simulink model "Mdl_Speed"  (R2024b)
settings: Solver=FixedStepDiscrete  StartTime=0.0  StopTime=10.0  FixedStep=0.1  RelTol=1e-3  EnableMultiTasking=on
values from neighbouring files (symbols this model uses):
  AI_TEMP_ADC_COUNT_1586 = mpt.Parameter    [Mdl_Speed_lookup.m]
  AI_TEMP_ADC_COUNT_1727 = mpt.Parameter    [Mdl_Speed_lookup.m]
  AI_TEMP_ADC_COUNT_1792 = mpt.Parameter    [Mdl_Speed_lookup.m]
  AI_TEMP_ADC_COUNT_1891 = mpt.Parameter    [Mdl_Speed_lookup.m]
  C_ADR = mpt.Parameter    [Mdl_Speed_lookup.m]
  C_CANADA = mpt.Parameter    [Mdl_Speed_lookup.m]
  C_EUROPE = mpt.Parameter    [Mdl_Speed_lookup.m]
  C_KOREA = mpt.Parameter    [Mdl_Speed_lookup.m]
  C_MEXICO = mpt.Parameter    [Mdl_Speed_lookup.m]
  C_UK = mpt.Parameter    [Mdl_Speed_lookup.m]
  C_USA = mpt.Parameter    [Mdl_Speed_lookup.m]
  eSP_ADR = mpt.Parameter    [Speed_Table_Type_param.m]
  eSP_CANADA = mpt.Parameter    [Speed_Table_Type_param.m]
  eSP_ECE = mpt.Parameter    [Speed_Table_Type_param.m]
  eSP_EUROPE = mpt.Parameter    [Speed_Table_Type_param.m]
  eSP_KOREA_FMVSS = mpt.Parameter    [Speed_Table_Type_param.m]
  eSP_KOREA_UN_R = mpt.Parameter    [Speed_Table_Type_param.m]
  eSP_MEXICO_FMVSS = mpt.Parameter    [Speed_Table_Type_param.m]
  eSP_MEXICO_UN_R = mpt.Parameter    [Speed_Table_Type_param.m]
  eSP_UK = mpt.Parameter    [Speed_Table_Type_param.m]
  eSP_USA = mpt.Parameter    [Speed_Table_Type_param.m]
  INDEX_MCUID0262 = mpt.Parameter    [Mdl_Speed_lookup.m]
  INDEX_MCUID0263 = mpt.Parameter    [Mdl_Speed_lookup.m]
  Initial_data = mpt.Parameter    [Mdl_Speed_lookup.m]
  MCUID0809 = mpt.Parameter    [Mdl_Speed_DD.m]
  MCUID0810 = mpt.Parameter    [Mdl_Speed_DD.m]
  MCUID_MAX_VAL = mpt.Parameter    [Mdl_Speed_lookup.m]
  MIN_SPEED_VALUE = mpt.Parameter    [Mdl_Speed_lookup.m]
  RESOLUTION_VAL_100 = mpt.Parameter    [Mdl_Speed_lookup.m]
  RESOLUTION_VAL_103 = mpt.Parameter    [Mdl_Speed_lookup.m]
  RESOLUTION_VAL_50 = mpt.Parameter    [Mdl_Speed_lookup.m]
  RESOLUTION_VAL_64 = mpt.Parameter    [Mdl_Speed_lookup.m]
  RESOLUTION_VAL_MINUS_100 = mpt.Parameter    [Mdl_Speed_lookup.m]
  SPEED_AVG_REF = mpt.Parameter    [Mdl_Speed_lookup.m]
  SPEED_CHECK_VALUE_ONE = mpt.Parameter    [Mdl_Speed_lookup.m]
  SPEED_UPDATE_0_28S = mpt.Parameter    [Mdl_Speed_lookup.m]
  SPEED_UPDATE_0_5S = mpt.Parameter    [Mdl_Speed_lookup.m]
  SPEED_UPDATE_1_5S = mpt.Parameter    [Mdl_Speed_lookup.m]
  SPEED_UPDATE_1S = mpt.Parameter    [Mdl_Speed_lookup.m]
  SPEED_ZERO = mpt.Parameter    [Mdl_Speed_lookup.m]
  VAL_ONE = mpt.Parameter    [Mdl_Speed_lookup.m]
  VAL_ZERO = mpt.Parameter    [Mdl_Speed_lookup.m]
undefined symbols (not defined in the file or in its folder): Arr_u8_100_type_instance, Arr_u8_1024_type_instance, Arr_u8_10_type_instance, Arr_u8_128_type_instance, Arr_u8_16_type_instance, Arr_u8_17_type_instance, Arr_u8_2048_type_instance, Arr_u8_256_type_instance, Arr_u8_32_type_instance, Arr_u8_3_type_instance, Arr_u8_46_type_instance, Arr_u8_48_type_instance, Arr_u8_61_type_instance, Arr_u8_64_type_instance, Arr_u8_8_type_instance, Arr_u8_9_type_instance, CLUSTER_ACTIVE, eIO_ADC_AI_TEMP_RTC, eSIGNAL_MISSING, eSIGNAL_NEVER_RECEIVED, eVehicleSpeedABSIn, IgnOff, IgnOn, IoHwAb_AdcSignalIdType_type_instance, IoHwAb_ErrorType_type_instance, pJustRcvdStatus, RxCan_SignalClearJustRcvdStatus, RxCan_SignalGetJustRcvdStatus, RxCan_SignalInvalidProcessingControl, RxCan_SignalMissingProcessingControl, RxCan_SignalNRProcessingControl, SignalId, SPEED_MAX_RESOLUTION, Status, tRxSignalId_type_instance, tRxSignalJustRcvdStatus_type_instance, tRxSignalStatus_type_instance
libraries: simulink x9
(part 2 of 3)

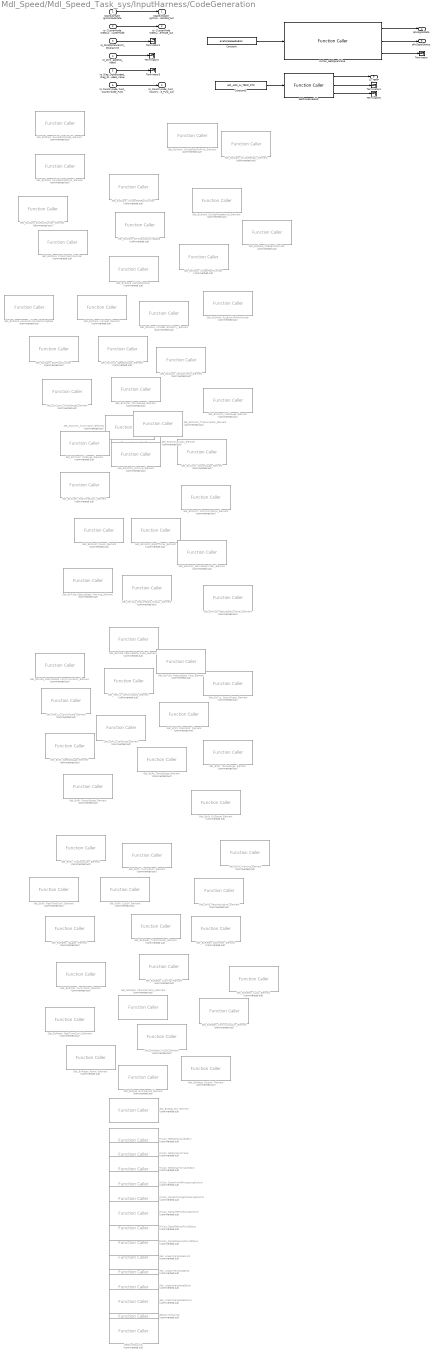
== system Mdl_Speed/Mdl_Speed_Task_sys/InputHarness/CodeGeneration ==
  rpIgnSubstate_IgnitionSubstate : Inport  OutDataTypeStr=IgntionSubstateType  PortDimensions=1
  rp_ClusterMode_WSSCurrentClusterMode : Inport  Port=2  OutDataTypeStr=ClusterModes  PortDimensions=1
  rp_DispDistanceUnit_DisplayUnit : Inport  Port=3  OutDataTypeStr=uint8  PortDimensions=1
  rp_Dcm_appStop_AppId : Inport  Port=4  OutDataTypeStr=IOCtrl_Type  PortDimensions=1
  rp_Diag_Digitalspeed_Diag_Digital_Speed_Value : Inport  Port=5  OutDataTypeStr=uint16  PortDimensions=1
  rp_Countrycode_Func_CountryCode_Func : Inport  Port=6  OutDataTypeStr=CountryCode_FuncType  PortDimensions=1
  Constant : Constant  Value=eVehicleSpeedABSIn
  Constant5 : Constant  Value=eIO_ADC_AI_TEMP_RTC  OutDataTypeStr=uint8
  GetAsyncRawAdc : FunctionCaller  Commented=on  FunctionPrototype=[AsyncRawAdc,ErrorStatus,error_status] = GetAsyncRawAdc(AdcId)  InputArgumentSpecifications=IoHwAb_AdcSignalIdType_type_instance(1)  OutputArgumentSpecifications=uint16(1) ,IoHwAb_ErrorType_type_instance(1) ,uint8(1)
  GetProcessedAdc : FunctionCaller  FunctionPrototype=[ProcessedAdc,ErrorStatus,error_status] = GetProcessedAdc(AdcId)  InputArgumentSpecifications=IoHwAb_AdcSignalIdType_type_instance(1)  OutputArgumentSpecifications=int32(1) ,IoHwAb_ErrorType_type_instance(1) ,uint8(1)
  GetSyncRawAdc : FunctionCaller  Commented=on  FunctionPrototype=[SyncRawAdc,ErrorStatus,error_status] = GetSyncRawAdc(AdcId)  InputArgumentSpecifications=IoHwAb_AdcSignalIdType_type_instance(1)  OutputArgumentSpecifications=uint16(1) ,IoHwAb_ErrorType_type_instance(1) ,uint8(1)
  Get_BsConst_Audio_Element : FunctionCaller  Commented=on  FunctionPrototype=[Ptr,error_status] = Get_BsConst_Audio_Element()  InputArgumentSpecifications=<Enter example>  OutputArgumentSpecifications=Arr_u8_128_type_instance(1) ,uint8(1)
  Get_BsConst_Communication_Element : FunctionCaller  Commented=on  FunctionPrototype=[Ptr,error_status] = Get_BsConst_Communication_Element()  InputArgumentSpecifications=<Enter example>  OutputArgumentSpecifications=Arr_u8_64_type_instance(1) ,uint8(1)
  Get_BsConst_EngOffTimer_Element : FunctionCaller  Commented=on  FunctionPrototype=[Ptr,error_status] = Get_BsConst_EngOffTimer_Element()  InputArgumentSpecifications=<Enter example>  OutputArgumentSpecifications=Arr_u8_32_type_instance(1) ,uint8(1)
  Get_BsConst_FuelGauge_Element : FunctionCaller  Commented=on  FunctionPrototype=[Ptr,error_status] = Get_BsConst_FuelGauge_Element()  InputArgumentSpecifications=<Enter example>  OutputArgumentSpecifications=Arr_u8_128_type_instance(1) ,uint8(1)
  Get_BsConst_Illumination_Element : FunctionCaller  Commented=on  FunctionPrototype=[Ptr,error_status] = Get_BsConst_Illumination_Element()  InputArgumentSpecifications=<Enter example>  OutputArgumentSpecifications=Arr_u8_128_type_instance(1) ,uint8(1)
  Get_BsConst_OilGauge_Element : FunctionCaller  Commented=on  FunctionPrototype=[Ptr,error_status] = Get_BsConst_OilGauge_Element()  InputArgumentSpecifications=<Enter example>  OutputArgumentSpecifications=Arr_u8_64_type_instance(1) ,uint8(1)
  Get_BsConst_PowerGauge_Element : FunctionCaller  Commented=on  FunctionPrototype=[Ptr,error_status] = Get_BsConst_PowerGauge_Element()  InputArgumentSpecifications=<Enter example>  OutputArgumentSpecifications=Arr_u8_64_type_instance(1) ,uint8(1)
  Get_BsConst_Power_Element : FunctionCaller  Commented=on  FunctionPrototype=[Ptr,error_status] = Get_BsConst_Power_Element()  InputArgumentSpecifications=<Enter example>  OutputArgumentSpecifications=Arr_u8_32_type_instance(1) ,uint8(1)
  Get_BsConst_RealTimeClock_Element : FunctionCaller  Commented=on  FunctionPrototype=[Ptr,error_status] = Get_BsConst_RealTimeClock_Element()  InputArgumentSpecifications=<Enter example>  OutputArgumentSpecifications=Arr_u8_48_type_instance(1) ,uint8(1)
  Get_BsConst_ServiceReminder_Element : FunctionCaller  Commented=on  FunctionPrototype=[Ptr,error_status] = Get_BsConst_ServiceReminder_Element()  InputArgumentSpecifications=<Enter example>  OutputArgumentSpecifications=Arr_u8_48_type_instance(1) ,uint8(1)
  Get_BsConst_SpeedoGauge_Element : FunctionCaller  Commented=on  FunctionPrototype=[Ptr,error_status] = Get_BsConst_SpeedoGauge_Element()  InputArgumentSpecifications=<Enter example>  OutputArgumentSpecifications=Arr_u8_64_type_instance(1) ,uint8(1)
  Get_BsConst_TachoGauge_Element : FunctionCaller  Commented=on  FunctionPrototype=[Ptr,error_status] = Get_BsConst_TachoGauge_Element()  InputArgumentSpecifications=<Enter example>  OutputArgumentSpecifications=Arr_u8_64_type_instance(1) ,uint8(1)
  Get_BsConst_TempGauge_Element : FunctionCaller  Commented=on  FunctionPrototype=[Ptr,error_status] = Get_BsConst_TempGauge_Element()  InputArgumentSpecifications=<Enter example>  OutputArgumentSpecifications=Arr_u8_64_type_instance(1) ,uint8(1)
  Get_BsConst_TripComputer_Element : FunctionCaller  Commented=on  FunctionPrototype=[Ptr,error_status] = Get_BsConst_TripComputer_Element()  InputArgumentSpecifications=<Enter example>  OutputArgumentSpecifications=Arr_u8_64_type_instance(1) ,uint8(1)
  Get_BsConst_Warning_Element : FunctionCaller  Commented=on  FunctionPrototype=[Ptr,error_status] = Get_BsConst_Warning_Element()  InputArgumentSpecifications=<Enter example>  OutputArgumentSpecifications=Arr_u8_64_type_instance(1) ,uint8(1)
  Get_BsCys_Certicificate_Element : FunctionCaller  Commented=on  FunctionPrototype=[Ptr,error_status] = Get_BsCys_Certicificate_Element()  InputArgumentSpecifications=<Enter example>  OutputArgumentSpecifications=Arr_u8_64_type_instance(1) ,uint8(1)
  Get_BsDiag_Dtc_Element : FunctionCaller  Commented=on  FunctionPrototype=[Ptr,error_status] = Get_BsDiag_Dtc_Element()  InputArgumentSpecifications=<Enter example>  OutputArgumentSpecifications=Arr_u8_2048_type_instance(1) ,uint8(1)
  Get_BsDiag_ErrorRecord_Element : FunctionCaller  Commented=on  FunctionPrototype=[Ptr,error_status] = Get_BsDiag_ErrorRecord_Element()  InputArgumentSpecifications=<Enter example>  OutputArgumentSpecifications=Arr_u8_1024_type_instance(1) ,uint8(1)
  Get_BsFuSa_FeatureData_Audio_Element : FunctionCaller  Commented=on  FunctionPrototype=[Ptr,error_status] = Get_BsFuSa_FeatureData_Audio_Element()  InputArgumentSpecifications=<Enter example>  OutputArgumentSpecifications=Arr_u8_8_type_instance(1) ,uint8(1)
  Get_BsFuSa_FeatureData_Communication_Element : FunctionCaller  Commented=on  FunctionPrototype=[Ptr,error_status] = Get_BsFuSa_FeatureData_Communication_Element()  InputArgumentSpecifications=<Enter example>  OutputArgumentSpecifications=Arr_u8_9_type_instance(1) ,uint8(1)
  Get_BsFuSa_FeatureData_Display_Element : FunctionCaller  Commented=on  FunctionPrototype=[Ptr,error_status] = Get_BsFuSa_FeatureData_Display_Element()  InputArgumentSpecifications=<Enter example>  OutputArgumentSpecifications=uint16(1) ,uint8(1)
  Get_BsFuSa_FeatureData_Fota_Element : FunctionCaller  Commented=on  FunctionPrototype=[Ptr,error_status] = Get_BsFuSa_FeatureData_Fota_Element()  InputArgumentSpecifications=<Enter example>  OutputArgumentSpecifications=uint16(1) ,uint8(1)
  Get_BsFuSa_FeatureData_Power_Element : FunctionCaller  Commented=on  FunctionPrototype=[Ptr,error_status] = Get_BsFuSa_FeatureData_Power_Element()  InputArgumentSpecifications=<Enter example>  OutputArgumentSpecifications=Arr_u8_10_type_instance(1) ,uint8(1)
  Get_BsFuSa_FeatureData_Warning_Element : FunctionCaller  Commented=on  FunctionPrototype=[Ptr,error_status] = Get_BsFuSa_FeatureData_Warning_Element()  InputArgumentSpecifications=<Enter example>  OutputArgumentSpecifications=Arr_u8_3_type_instance(1) ,uint8(1)
  Get_BsReten_Audio_Element : FunctionCaller  Commented=on  FunctionPrototype=[Ptr,error_status] = Get_BsReten_Audio_Element()  InputArgumentSpecifications=<Enter example>  OutputArgumentSpecifications=Arr_u8_100_type_instance(1) ,uint8(1)
  Get_BsReten_Communication_Element : FunctionCaller  Commented=on  FunctionPrototype=[Ptr,error_status] = Get_BsReten_Communication_Element()  InputArgumentSpecifications=<Enter example>  OutputArgumentSpecifications=Arr_u8_100_type_instance(1) ,uint8(1)
  Get_BsReten_Display_Element : FunctionCaller  Commented=on  FunctionPrototype=[Ptr,error_status] = Get_BsReten_Display_Element()  InputArgumentSpecifications=<Enter example>  OutputArgumentSpecifications=Arr_u8_100_type_instance(1) ,uint8(1)
  Get_BsReten_Gauges_Element : FunctionCaller  Commented=on  FunctionPrototype=[Ptr,error_status] = Get_BsReten_Gauges_Element()  InputArgumentSpecifications=<Enter example>  OutputArgumentSpecifications=Arr_u8_100_type_instance(1) ,uint8(1)
  Get_BsReten_Illumination_Element : FunctionCaller  Commented=on  FunctionPrototype=[Ptr,error_status] = Get_BsReten_Illumination_Element()  InputArgumentSpecifications=<Enter example>  OutputArgumentSpecifications=Arr_u8_100_type_instance(1) ,uint8(1)
  Get_BsReten_Odometer_Element : FunctionCaller  Commented=on  FunctionPrototype=[Ptr,error_status] = Get_BsReten_Odometer_Element()  InputArgumentSpecifications=<Enter example>  OutputArgumentSpecifications=Arr_u8_100_type_instance(1) ,uint8(1)
  Get_BsReten_Personalization_Element : FunctionCaller  Commented=on  FunctionPrototype=[Ptr,error_status] = Get_BsReten_Personalization_Element()  InputArgumentSpecifications=<Enter example>  OutputArgumentSpecifications=Arr_u8_100_type_instance(1) ,uint8(1)
  Get_BsReten_Power_Element : FunctionCaller  Commented=on  FunctionPrototype=[Ptr,error_status] = Get_BsReten_Power_Element()  InputArgumentSpecifications=<Enter example>  OutputArgumentSpecifications=Arr_u8_100_type_instance(1) ,uint8(1)
  Get_BsReten_RealTimeClock_Element : FunctionCaller  Commented=on  FunctionPrototype=[Ptr,error_status] = Get_BsReten_RealTimeClock_Element()  InputArgumentSpecifications=<Enter example>  OutputArgumentSpecifications=Arr_u8_100_type_instance(1) ,uint8(1)
  Get_BsReten_Tripcomputer_Element : FunctionCaller  Commented=on  FunctionPrototype=[Ptr,error_status] = Get_BsReten_Tripcomputer_Element()  InputArgumentSpecifications=<Enter example>  OutputArgumentSpecifications=Arr_u8_100_type_instance(1) ,uint8(1)
  Get_BsReten_VisDlt_Element : FunctionCaller  Commented=on  FunctionPrototype=[Ptr,error_status] = Get_BsReten_VisDlt_Element()  InputArgumentSpecifications=<Enter example>  OutputArgumentSpecifications=Arr_u8_256_type_instance(1) ,uint8(1)
  Get_BsReten_Warning_Element : FunctionCaller  Commented=on  FunctionPrototype=[Ptr,error_status] = Get_BsReten_Warning_Element()  InputArgumentSpecifications=<Enter example>  OutputArgumentSpecifications=Arr_u8_100_type_instance(1) ,uint8(1)
  Get_BsRt_CusDlt_Element : FunctionCaller  Commented=on  FunctionPrototype=[Ptr,error_status] = Get_BsRt_CusDlt_Element()  InputArgumentSpecifications=<Enter example>  OutputArgumentSpecifications=Arr_u8_128_type_instance(1) ,uint8(1)
  Get_BsRt_FuelGauge_Element : FunctionCaller  Commented=on  FunctionPrototype=[Ptr,error_status] = Get_BsRt_FuelGauge_Element()  InputArgumentSpecifications=<Enter example>  OutputArgumentSpecifications=Arr_u8_32_type_instance(1) ,uint8(1)
  Get_BsRt_Illumination_Element : FunctionCaller  Commented=on  FunctionPrototype=[Ptr,error_status] = Get_BsRt_Illumination_Element()  InputArgumentSpecifications=<Enter example>  OutputArgumentSpecifications=Arr_u8_100_type_instance(1) ,uint8(1)
  Get_BsRt_Odometer_Element : FunctionCaller  Commented=on  FunctionPrototype=[Ptr,error_status] = Get_BsRt_Odometer_Element()  InputArgumentSpecifications=<Enter example>  OutputArgumentSpecifications=Arr_u8_128_type_instance(1) ,uint8(1)
  Get_BsRt_OilGauge_Element : FunctionCaller  Commented=on  FunctionPrototype=[Ptr,error_status] = Get_BsRt_OilGauge_Element()  InputArgumentSpecifications=<Enter example>  OutputArgumentSpecifications=Arr_u8_8_type_instance(1) ,uint8(1)
  Get_BsRt_Personalization_Element : FunctionCaller  Commented=on  FunctionPrototype=[Ptr,error_status] = Get_BsRt_Personalization_Element()  InputArgumentSpecifications=<Enter example>  OutputArgumentSpecifications=Arr_u8_128_type_instance(1) ,uint8(1)
  Get_BsRt_PowerGauge_Element : FunctionCaller  Commented=on  FunctionPrototype=[Ptr,error_status] = Get_BsRt_PowerGauge_Element()  InputArgumentSpecifications=<Enter example>  OutputArgumentSpecifications=Arr_u8_32_type_instance(1) ,uint8(1)
  Get_BsRt_RealTimeClock_Element : FunctionCaller  Commented=on  FunctionPrototype=[Ptr,error_status] = Get_BsRt_RealTimeClock_Element()  InputArgumentSpecifications=<Enter example>  OutputArgumentSpecifications=Arr_u8_48_type_instance(1) ,uint8(1)
  Get_BsRt_SpeedoGauge_Element : FunctionCaller  Commented=on  FunctionPrototype=[Ptr,error_status] = Get_BsRt_SpeedoGauge_Element()  InputArgumentSpecifications=<Enter example>  OutputArgumentSpecifications=Arr_u8_8_type_instance(1) ,uint8(1)
  Get_BsRt_TachoGauge_Element : FunctionCaller  Commented=on  FunctionPrototype=[Ptr,error_status] = Get_BsRt_TachoGauge_Element()  InputArgumentSpecifications=<Enter example>  OutputArgumentSpecifications=Arr_u8_16_type_instance(1) ,uint8(1)
  Get_BsRt_TempGauge_Element : FunctionCaller  Commented=on  FunctionPrototype=[Ptr,error_status] = Get_BsRt_TempGauge_Element()  InputArgumentSpecifications=<Enter example>  OutputArgumentSpecifications=Arr_u8_32_type_instance(1) ,uint8(1)
  Get_BsRt_TripComputer_Element : FunctionCaller  Commented=on  FunctionPrototype=[Ptr,error_status] = Get_BsRt_TripComputer_Element()  InputArgumentSpecifications=<Enter example>  OutputArgumentSpecifications=Arr_u8_64_type_instance(1) ,uint8(1)
  Get_BsRt_Warning_Element : FunctionCaller  Commented=on  FunctionPrototype=[Ptr,error_status] = Get_BsRt_Warning_Element()  InputArgumentSpecifications=<Enter example>  OutputArgumentSpecifications=Arr_u8_32_type_instance(1) ,uint8(1)
  Get_BsShare_AssemblyManufacturingDate : FunctionCaller  Commented=on  FunctionPrototype=[Ptr,error_status] = Get_BsShare_AssemblyManufacturingDate()  InputArgumentSpecifications=<Enter example>  OutputArgumentSpecifications=Arr_u8_3_type_instance(1) ,uint8(1)
  Get_BsShare_AssemblyPlantNumber : FunctionCaller  Commented=on  FunctionPrototype=[Ptr,error_status] = Get_BsShare_AssemblyPlantNumber()  InputArgumentSpecifications=<Enter example>  OutputArgumentSpecifications=Arr_u8_3_type_instance(1) ,uint8(1)
  Get_BsShare_EcuPartNumber_Element : FunctionCaller  Commented=on  FunctionPrototype=[Ptr,error_status] = Get_BsShare_EcuPartNumber_Element()  InputArgumentSpecifications=<Enter example>  OutputArgumentSpecifications=Arr_u8_61_type_instance(1) ,uint8(1)
  Get_BsShare_HWModification : FunctionCaller  Commented=on  FunctionPrototype=[Ptr,error_status] = Get_BsShare_HWModification()  InputArgumentSpecifications=<Enter example>  OutputArgumentSpecifications=uint16(1) ,uint8(1)
  Get_BsShare_PCBSerialNumber : FunctionCaller  Commented=on  FunctionPrototype=[Ptr,error_status] = Get_BsShare_PCBSerialNumber()  InputArgumentSpecifications=<Enter example>  OutputArgumentSpecifications=Arr_u8_9_type_instance(1) ,uint8(1)
  Get_BsShare_ProductSerialNumber : FunctionCaller  Commented=on  FunctionPrototype=[Ptr,error_status] = Get_BsShare_ProductSerialNumber()  InputArgumentSpecifications=<Enter example>  OutputArgumentSpecifications=Arr_u8_10_type_instance(1) ,uint8(1)
  Get_BsShare_SMTManufacturingDate : FunctionCaller  Commented=on  FunctionPrototype=[Ptr,error_status] = Get_BsShare_SMTManufacturingDate()  InputArgumentSpecifications=<Enter example>  OutputArgumentSpecifications=Arr_u8_3_type_instance(1) ,uint8(1)
  Get_BsShare_SMTPlantNumber : FunctionCaller  Commented=on  FunctionPrototype=[Ptr,error_status] = Get_BsShare_SMTPlantNumber()  InputArgumentSpecifications=<Enter example>  OutputArgumentSpecifications=Arr_u8_3_type_instance(1) ,uint8(1)
  Get_BsShare_SwUpdFotaFinPrint_Element : FunctionCaller  Commented=on  FunctionPrototype=[Ptr,error_status] = Get_BsShare_SwUpdFotaFinPrint_Element()  InputArgumentSpecifications=<Enter example>  OutputArgumentSpecifications=Arr_u8_32_type_instance(1) ,uint8(1)
  Get_BsShare_SwUpdFotaMode_Element : FunctionCaller  Commented=on  FunctionPrototype=[Ptr,error_status] = Get_BsShare_SwUpdFotaMode_Element()  InputArgumentSpecifications=<Enter example>  OutputArgumentSpecifications=Arr_u8_16_type_instance(1) ,uint8(1)
  Get_BsShare_SwUpdFotaStatus_Element : FunctionCaller  Commented=on  FunctionPrototype=[Ptr,error_status] = Get_BsShare_SwUpdFotaStatus_Element()  InputArgumentSpecifications=<Enter example>  OutputArgumentSpecifications=Arr_u8_48_type_instance(1) ,uint8(1)
  Get_BsShare_SwUpdFotadecrypt_Element : FunctionCaller  Commented=on  FunctionPrototype=[Ptr,error_status] = Get_BsShare_SwUpdFotadecrypt_Element()  InputArgumentSpecifications=<Enter example>  OutputArgumentSpecifications=Arr_u8_64_type_instance(1) ,uint8(1)
  Get_BsShare_SwUpdReflash_Element : FunctionCaller  Commented=on  FunctionPrototype=[Ptr,error_status] = Get_BsShare_SwUpdReflash_Element()  InputArgumentSpecifications=<Enter example>  OutputArgumentSpecifications=Arr_u8_8_type_instance(1) ,uint8(1)
  Get_BsShare_VehicleConfig_Element : FunctionCaller  Commented=on  FunctionPrototype=[Ptr,error_status] = Get_BsShare_VehicleConfig_Element()  InputArgumentSpecifications=<Enter example>  OutputArgumentSpecifications=Arr_u8_256_type_instance(1) ,uint8(1)
  Get_BsShare_VisMeet_EOLEntry_Element : FunctionCaller  Commented=on  FunctionPrototype=[Ptr,error_status] = Get_BsShare_VisMeet_EOLEntry_Element()  InputArgumentSpecifications=<Enter example>  OutputArgumentSpecifications=uint16(1) ,uint8(1)
  Get_BsShare_VisMeet_Element : FunctionCaller  Commented=on  FunctionPrototype=[Ptr,error_status] = Get_BsShare_VisMeet_Element()  InputArgumentSpecifications=<Enter example>  OutputArgumentSpecifications=Arr_u8_46_type_instance(1) ,uint8(1)
  Get_BsShare_VisteonPCBPartNumber : FunctionCaller  Commented=on  FunctionPrototype=[Ptr,error_status] = Get_BsShare_VisteonPCBPartNumber()  InputArgumentSpecifications=<Enter example>  OutputArgumentSpecifications=Arr_u8_17_type_instance(1) ,uint8(1)
  Get_BsShare_VisteonPartNumber : FunctionCaller  Commented=on  FunctionPrototype=[Ptr,error_status] = Get_BsShare_VisteonPartNumber()  InputArgumentSpecifications=<Enter example>  OutputArgumentSpecifications=Arr_u8_17_type_instance(1) ,uint8(1)
  Get_LinearInterpolateByte : FunctionCaller  Commented=on  FunctionPrototype=[ptr_table,Ptr_Lin_Return] = Get_LinearInterpolateByte(lookupvalue)  InputArgumentSpecifications=uint8(1)  OutputArgumentSpecifications=uint8(1) ,uint8(1)
  Get_LinearInterpolateSByte : FunctionCaller  Commented=on  FunctionPrototype=[ptr_table,Ptr_Lin_Return] = Get_LinearInterpolateSByte(lookupvalue)  InputArgumentSpecifications=int8(1)  OutputArgumentSpecifications=int8(1) ,int8(1)
  Get_LinearInterpolateSWord : FunctionCaller  Commented=on  FunctionPrototype=[ptr_table,Ptr_Lin_Return] = Get_LinearInterpolateSWord(lookupvalue)  InputArgumentSpecifications=int16(1)  OutputArgumentSpecifications=int16(1) ,int16(1)
  Get_LinearInterpolateWord : FunctionCaller  Commented=on  FunctionPrototype=[ptr_table,Ptr_Lin_Return] = Get_LinearInterpolateWord(lookupvalue)  InputArgumentSpecifications=uint16(1)  OutputArgumentSpecifications=uint16(1) ,uint16(1)
  Get_RefCys_Certicificate1_Element : FunctionCaller  Commented=on  FunctionPrototype=[Ptr,error_status] = Get_RefCys_Certicificate1_Element()  InputArgumentSpecifications=<Enter example>  OutputArgumentSpecifications=Arr_u8_64_type_instance(1) ,uint8(1)
  Get_RefCys_Certicificate_Element : FunctionCaller  Commented=on  FunctionPrototype=[Ptr,error_status] = Get_RefCys_Certicificate_Element()  InputArgumentSpecifications=<Enter example>  OutputArgumentSpecifications=Arr_u8_64_type_instance(1) ,uint8(1)
  RxCan_GetSignalValue : FunctionCaller  FunctionPrototype=[pSignalValue,pSignalStatus,error_status] = RxCan_GetSignalValue(SignalId)  InputArgumentSpecifications=tRxSignalId_type_instance(1)  OutputArgumentSpecifications=uint8(1) ,tRxSignalStatus_type_instance(1) ,uint8(1)
  RxCan_GetSignalValueU8Arr : FunctionCaller  Commented=on  FunctionPrototype=[pSignalValue,pSignalStatus,pSignalLength,error_status] = RxCan_GetSignalValueU8Arr(SignalId)  InputArgumentSpecifications=tRxSignalId_type_instance(1)  OutputArgumentSpecifications=uint8(1) ,tRxSignalStatus_type_instance(1) ,uint32(1) ,uint8(1)
  RxCan_SetSignalInitValue : FunctionCaller  Commented=on  FunctionPrototype=[pSignalValue,error_status] = RxCan_SetSignalInitValue(SignalId)  InputArgumentSpecifications=tRxSignalId_type_instance(1)  OutputArgumentSpecifications=uint8(1) ,uint8(1)
  RxCan_SetSignalInitValueU8Arr : FunctionCaller  Commented=on  FunctionPrototype=[pSignaValue,pSignalLength,error_status] = RxCan_SetSignalInitValueU8Arr(SignalId)  InputArgumentSpecifications=tRxSignalId_type_instance(1)  OutputArgumentSpecifications=uint8(1) ,uint32(1) ,uint8(1)
  RxCan_SignalClearJustRcvdStatus : FunctionCaller  Commented=on  FunctionPrototype=RxCan_SignalClearJustRcvdStatus(SignalId)  InputArgumentSpecifications=tRxSignalId_type_instance(1)  OutputArgumentSpecifications=<Enter example>
  RxCan_SignalGetJustRcvdStatus : FunctionCaller  Commented=on  FunctionPrototype=RxCan_SignalGetJustRcvdStatus(SignalId,pJustRcvdStatus)  InputArgumentSpecifications=tRxSignalId_type_instance(1) ,tRxSignalJustRcvdStatus_type_instance(1)  OutputArgumentSpecifications=<Enter example>
  RxCan_SignalInvalidProcessingControl : FunctionCaller  Commented=on  FunctionPrototype=RxCan_SignalInvalidProcessingControl(SignalId,Status)  InputArgumentSpecifications=tRxSignalId_type_instance(1) ,boolean(1)  OutputArgumentSpecifications=<Enter example>
  RxCan_SignalMissingProcessingControl : FunctionCaller  Commented=on  FunctionPrototype=RxCan_SignalMissingProcessingControl(SignalId,Status)  InputArgumentSpecifications=tRxSignalId_type_instance(1) ,boolean(1)  OutputArgumentSpecifications=<Enter example>
  RxCan_SignalNRProcessingControl : FunctionCaller  Commented=on  FunctionPrototype=RxCan_SignalNRProcessingControl(SignalId,Status)  InputArgumentSpecifications=tRxSignalId_type_instance(1) ,boolean(1)  OutputArgumentSpecifications=<Enter example>
  Terminator{,1..5} (6 alike) : Terminator
  rpIgnSubstate_IgnitionSubstate_out : Outport  OutDataTypeStr=IgntionSubstateType  PortDimensions=1
  rp_ClusterMode_WSSCurrentClusterMode_out : Outport  Port=2  OutDataTypeStr=ClusterModes  PortDimensions=1
  rp_Countrycode_Func_CountryCode_Func_out : Outport  Port=3  OutDataTypeStr=CountryCode_FuncType  PortDimensions=1
  pRxSignalData : Outport  Port=4  OutDataTypeStr=uint8  VectorParamsAs1DForOutWhenUnconnected=off
  pRxSignalStatus : Outport  Port=5  OutDataTypeStr=uint8  VectorParamsAs1DForOutWhenUnconnected=off
  AI_TEMP : Outport  Port=6  VectorParamsAs1DForOutWhenUnconnected=off
  wires:
  rpIgnSubstate_IgnitionSubstate/1 -> rpIgnSubstate_IgnitionSubstate_out/1
  rp_ClusterMode_WSSCurrentClusterMode/1 -> rp_ClusterMode_WSSCurrentClusterMode_out/1
  rp_Countrycode_Func_CountryCode_Func/1 -> rp_Countrycode_Func_CountryCode_Func_out/1
  Constant/1 -> RxCan_GetSignalValue/1
  RxCan_GetSignalValue/2 -> pRxSignalStatus/1
  RxCan_GetSignalValue/1 -> pRxSignalData/1
  RxCan_GetSignalValue/3 -> Terminator/1
  rp_DispDistanceUnit_DisplayUnit/1 -> Terminator1/1
  rp_Dcm_appStop_AppId/1 -> Terminator2/1
  rp_Diag_Digitalspeed_Diag_Digital_Speed_Value/1 -> Terminator3/1
  Constant5/1 -> GetProcessedAdc/1
  GetProcessedAdc/1 -> AI_TEMP/1
  GetProcessedAdc/2 -> Terminator4/1
  GetProcessedAdc/3 -> Terminator5/1

== system Mdl_Speed/Mdl_Speed_Task_sys/InputHarness/Simulation ==

== system Mdl_Speed/Mdl_Speed_Task_sys/OutputHarness/CodeGeneration ==
  pp_SPD_SP1_In_Status_SP1_In_Status_in : Inport  OutDataTypeStr=uint16  PortDimensions=1
  pp_SPD_Target_Status_Spd_Target_Status_in : Inport  Port=2  OutDataTypeStr=uint16  PortDimensions=1
  pp_SPD_Trim_Status_Spd_Trim_Status_in : Inport  Port=3  OutDataTypeStr=uint16  PortDimensions=1
  pp_SPD_Target2_Status_Spd_Target2_Status_in : Inport  Port=4  OutDataTypeStr=uint16  PortDimensions=1
  pp_SPD_Trim2_Status_Spd_Trim2_Status_in : Inport  Port=5  OutDataTypeStr=uint16  PortDimensions=1
  pp_SPD_Selection_Table_Speed_Selection_Table_in : Inport  Port=6  OutDataTypeStr=uint8  PortDimensions=1
  pp_SPD_SP1_In_Status_SP1_In_Status : Outport  OutDataTypeStr=uint16  PortDimensions=1
  pp_SPD_Target_Status_Spd_Target_Status : Outport  Port=2  OutDataTypeStr=uint16  PortDimensions=1
  pp_SPD_Trim_Status_Spd_Trim_Status : Outport  Port=3  OutDataTypeStr=uint16  PortDimensions=1
  pp_SPD_Target2_Status_Spd_Target2_Status : Outport  Port=4  OutDataTypeStr=uint16  PortDimensions=1
  pp_SPD_Trim2_Status_Spd_Trim2_Status : Outport  Port=5  OutDataTypeStr=uint16  PortDimensions=1
  pp_SPD_Selection_Table_Speed_Selection_Table : Outport  Port=6  OutDataTypeStr=uint8  PortDimensions=1
  wires:
  pp_SPD_Target2_Status_Spd_Target2_Status_in/1 -> pp_SPD_Target2_Status_Spd_Target2_Status/1
  pp_SPD_Trim2_Status_Spd_Trim2_Status_in/1 -> pp_SPD_Trim2_Status_Spd_Trim2_Status/1
  pp_SPD_Selection_Table_Speed_Selection_Table_in/1 -> pp_SPD_Selection_Table_Speed_Selection_Table/1
  pp_SPD_SP1_In_Status_SP1_In_Status_in/1 -> pp_SPD_SP1_In_Status_SP1_In_Status/1
  pp_SPD_Trim_Status_Spd_Trim_Status_in/1 -> pp_SPD_Trim_Status_Spd_Trim_Status/1
  pp_SPD_Target_Status_Spd_Target_Status_in/1 -> pp_SPD_Target_Status_Spd_Target_Status/1

== system Mdl_Speed/Mdl_Speed_Task_sys/OutputHarness/Simulation ==
  pp_SPD_SP1_In_Status_SP1_In_Status : Outport  OutDataTypeStr=uint16  PortDimensions=1
  pp_SPD_Target_Status_Spd_Target_Status : Outport  Port=2  OutDataTypeStr=uint16  PortDimensions=1
  pp_SPD_Trim_Status_Spd_Trim_Status : Outport  Port=3  OutDataTypeStr=uint16  PortDimensions=1
  pp_SPD_Target2_Status_Spd_Target2_Status : Outport  Port=4  OutDataTypeStr=uint16  PortDimensions=1
  pp_SPD_Trim2_Status_Spd_Trim2_Status : Outport  Port=5  OutDataTypeStr=uint16  PortDimensions=1
  pp_SPD_Selection_Table_Speed_Selection_Table : Outport  Port=6  OutDataTypeStr=uint8  PortDimensions=1

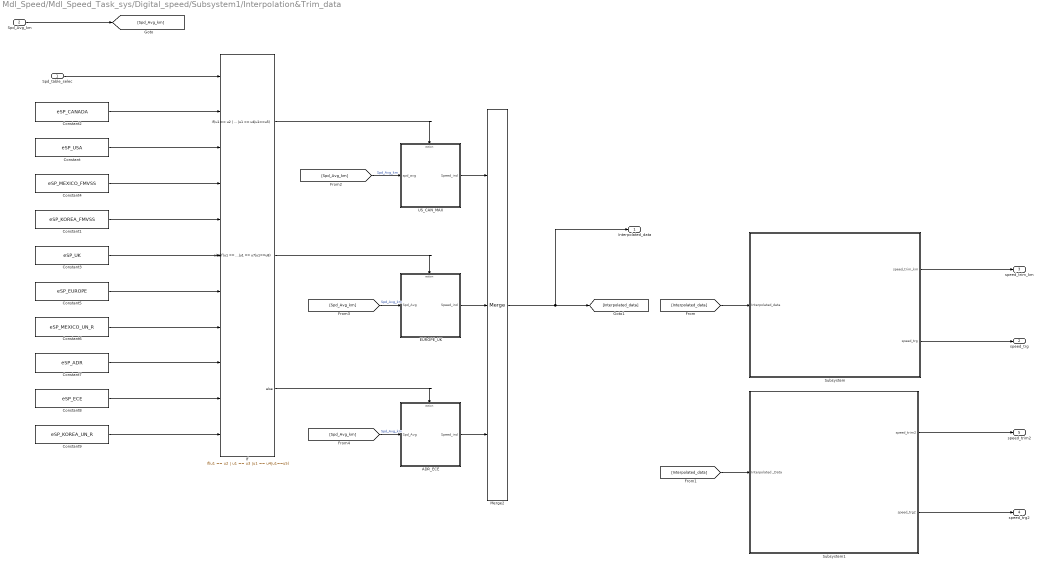
== system Mdl_Speed/Mdl_Speed_Task_sys/Digital_speed/Subsystem1/Interpolation&Trim_data ==
  Spd_table_selec : Inport
  Spd_Avg_km : Inport  Port=2
  ADR_ECE : Subsystem  TreatAsAtomicUnit=on
  Constant : Constant  Value=eSP_USA  OutDataTypeStr=uint8
  Constant1 : Constant  Value=eSP_KOREA_FMVSS  OutDataTypeStr=uint8
  Constant2 : Constant  Value=eSP_CANADA  OutDataTypeStr=uint8
  Constant3 : Constant  Value=eSP_UK  OutDataTypeStr=uint8
  Constant4 : Constant  Value=eSP_MEXICO_FMVSS  OutDataTypeStr=uint8
  Constant5 : Constant  Value=eSP_EUROPE  OutDataTypeStr=uint8
  Constant6 : Constant  Value=eSP_MEXICO_UN_R  OutDataTypeStr=uint8
  Constant7 : Constant  Value=eSP_ADR  OutDataTypeStr=uint8
  Constant8 : Constant  Value=eSP_ECE  OutDataTypeStr=uint8
  Constant9 : Constant  Value=eSP_KOREA_UN_R  OutDataTypeStr=uint8
  EUROPE_UK : Subsystem  TreatAsAtomicUnit=on
  If : If  NumInputs=11  IfExpression=u1 == u2 | u1 == u3 |u1 == u4|u1==u5  ElseIfExpressions=u1 == u6|u1 == u7|u1==u8
  Merge2 : Merge  Inputs=3
  Subsystem : Subsystem
  Subsystem1 : Subsystem
  US_CAN_MAX : Subsystem
  Interpolated_data : Outport  VectorParamsAs1DForOutWhenUnconnected=off
  speed_trg : Outport  Port=2  OutDataTypeStr=uint16  VectorParamsAs1DForOutWhenUnconnected=off
  speed_trim_km : Outport  Port=3  OutDataTypeStr=uint16  VectorParamsAs1DForOutWhenUnconnected=off
  speed_trg2 : Outport  Port=4  OutDataTypeStr=uint16  VectorParamsAs1DForOutWhenUnconnected=off
  speed_trim2 : Outport  Port=5  OutDataTypeStr=uint16  VectorParamsAs1DForOutWhenUnconnected=off
  wires:
  [Spd_Avg_km] -> US_CAN_MAX/1(spd_avg)  "Spd_Avg_km"
  [Spd_Avg_km] -> EUROPE_UK/1(Spd_Avg)  "Spd_Avg_km"
  [Spd_Avg_km] -> ADR_ECE/1(Spd_Avg)  "Spd_Avg_km"
  US_CAN_MAX/1(Speed_ind) -> Merge2/1
  Spd_Avg_km/1 -> [Spd_Avg_km]
  If/1 -> US_CAN_MAX/Action
  If/2 -> EUROPE_UK/Action
  EUROPE_UK/1(Speed_ind) -> Merge2/2
  ADR_ECE/1(Speed_ind) -> Merge2/3
  If/3 -> ADR_ECE/Action
  Constant2/1 -> If/2
  Constant1/1 -> If/5
  Constant/1 -> If/3
  Constant4/1 -> If/4
  Constant3/1 -> If/6
  Spd_table_selec/1 -> If/1
  Subsystem/1(speed_trim_km) -> speed_trim_km/1
  Subsystem/2(speed_trg) -> speed_trg/1
  Subsystem1/2(speed_trg2) -> speed_trg2/1
  Subsystem1/1(speed_trim2) -> speed_trim2/1
  Merge2/1 -> [Interpolated_data], Interpolated_data/1
  [Interpolated_data] -> Subsystem/1(Interpolated_data)
  [Interpolated_data] -> Subsystem1/1(Interpolated _Data)
  Constant5/1 -> If/7
  Constant6/1 -> If/8
  Constant7/1 -> If/9
  Constant8/1 -> If/10
  Constant9/1 -> If/11

== system Mdl_Speed/Mdl_Speed_Task_sys/Digital_speed/Subsystem1/SpeedTable_Selection ==
  CountrycodeFunc : Inport
  Constant : Constant  Value=MCUID0809
  Constant1 : Constant  Value=MCUID0810
  Truth Table : Truth Table  TreatAsAtomicUnit=on
  SpeedTable_Selec : Outport  VectorParamsAs1DForOutWhenUnconnected=off
  wires:
  CountrycodeFunc/1 -> Truth Table/1(Country_code_func)
  Truth Table/1(spd_selector) -> SpeedTable_Selec/1
  Constant/1 -> Truth Table/2(MCUID_0809)
  Constant1/1 -> Truth Table/3(MCUID_0810)

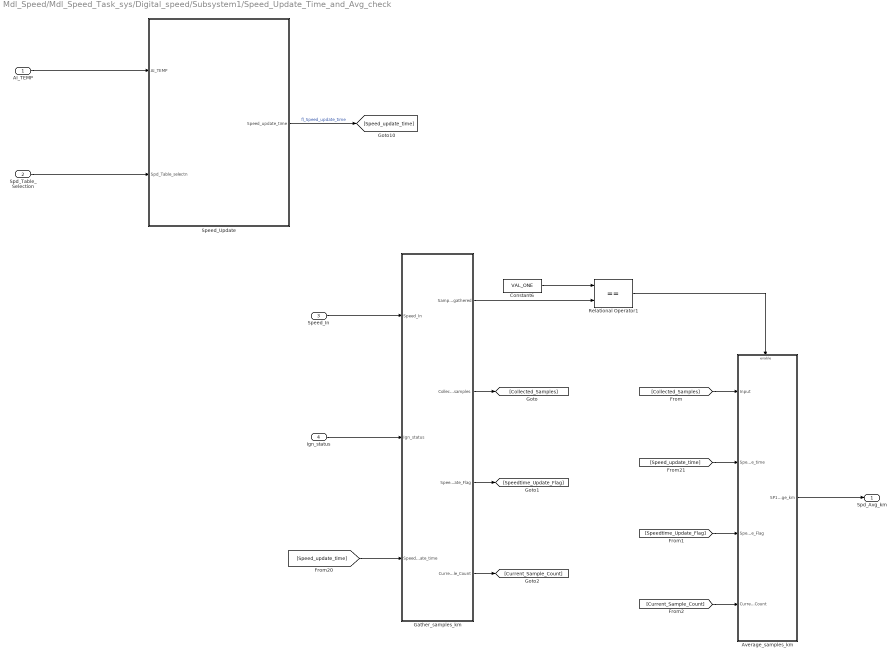
== system Mdl_Speed/Mdl_Speed_Task_sys/Digital_speed/Subsystem1/Speed_Update_Time_and_Avg_check ==
  AI_TEMP : Inport
  Spd_Table_Selection : Inport  Port=2
  Speed_In : Inport  Port=3
  Ign_status : Inport  Port=4
  Average_samples_km : Subsystem
  Constant6 : Constant  Value=VAL_ONE  OutDataTypeStr=uint8
  Gather_samples_km : Subsystem
  Relational Operator1 : RelationalOperator  Operator===  OutDataTypeStr=boolean  RndMeth=Simplest  InputSameDT=off
  Speed_Update : Truth Table  TreatAsAtomicUnit=on
  Spd_Avg_km : Outport  VectorParamsAs1DForOutWhenUnconnected=off
  wires:
  Average_samples_km/1(SP1_Average_km) -> Spd_Avg_km/1
  [Speed_update_time] -> Gather_samples_km/3(Speed_update_time)
  [Speed_update_time] -> Average_samples_km/2(Speed_update_time)
  Speed_Update/1(Speed_update_time) -> [Speed_update_time]  "fl_Speed_update_time"
  Gather_samples_km/1(Samples_gathered) -> Relational Operator1/2
  Relational Operator1/1 -> Average_samples_km/Enable
  Constant6/1 -> Relational Operator1/1
  Ign_status/1 -> Gather_samples_km/2(Ign_status)
  Speed_In/1 -> Gather_samples_km/1(Speed_In)
  AI_TEMP/1 -> Speed_Update/1(AI_TEMP)
  Gather_samples_km/2(Collect_samples) -> [Collected_Samples]
  Gather_samples_km/3(Speedtime_Update_Flag) -> [Speedtime_Update_Flag]
  Gather_samples_km/4(Current_Sample_Count) -> [Current_Sample_Count]
  [Collected_Samples] -> Average_samples_km/1(Input)
  [Speedtime_Update_Flag] -> Average_samples_km/3(Speedtime_Update_Flag)
  [Current_Sample_Count] -> Average_samples_km/4(Current_Sample_Count)
  Spd_Table_Selection/1 -> Speed_Update/2(Spd_Table_selectn)

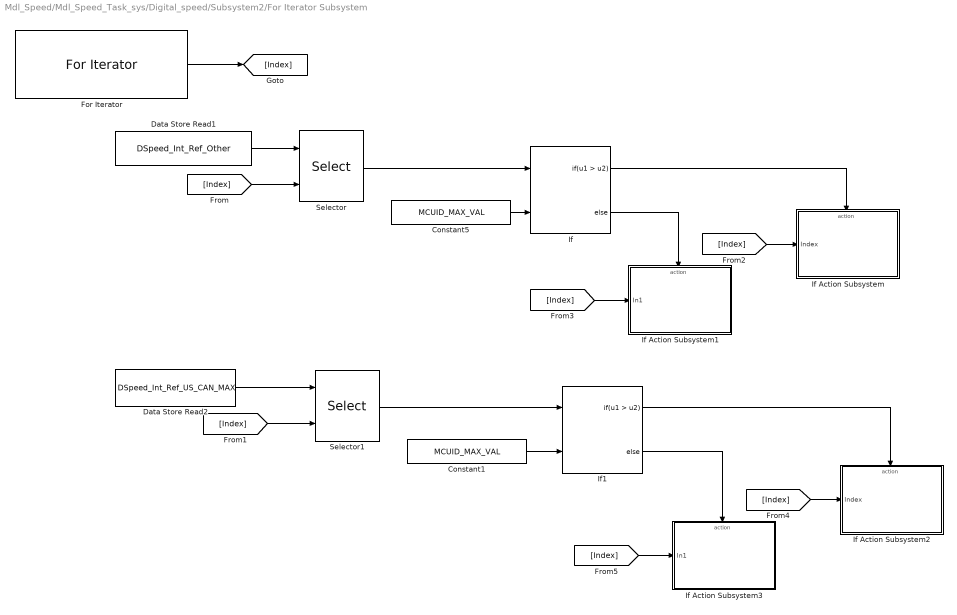
== system Mdl_Speed/Mdl_Speed_Task_sys/Digital_speed/Subsystem2/For Iterator Subsystem ==
  Constant1 : Constant  Value=MCUID_MAX_VAL
  Constant5 : Constant  Value=MCUID_MAX_VAL
  Data Store Read1 : DataStoreRead  DataStoreName=DSpeed_Int_Ref_Other  IndexOptions=Index vector (dialog)  Indices=1  OutputSizes=1
  Data Store Read2 : DataStoreRead  DataStoreName=DSpeed_Int_Ref_US_CAN_MAX  IndexOptions=Index vector (dialog)  Indices=1  OutputSizes=1
  For Iterator : ForIterator  ResetStates=reset  IterationLimit=21  IndexMode=Zero-based  IterationVariableDataType=int8
  If : If  NumInputs=2  IfExpression=u1 > u2
  If Action Subsystem : Subsystem  TreatAsAtomicUnit=on
  If Action Subsystem1 : Subsystem  TreatAsAtomicUnit=on
  If Action Subsystem2 : Subsystem  TreatAsAtomicUnit=on
  If Action Subsystem3 : Subsystem  TreatAsAtomicUnit=on
  If1 : If  NumInputs=2  IfExpression=u1 > u2
  Selector : Selector  IndexMode=Zero-based  InputPortWidth=21  IndexOptions=Index vector (port)  Indices=[1 3]  OutputSizes=1
  Selector1 : Selector  IndexMode=Zero-based  InputPortWidth=21  IndexOptions=Index vector (port)  Indices=[1 3]  OutputSizes=1
  wires:
  For Iterator/1 -> [Index]
  Data Store Read1/1 -> Selector/1
  [Index] -> Selector/2
  [Index] -> Selector1/2
  Data Store Read2/1 -> Selector1/1
  Constant5/1 -> If/2
  Selector/1 -> If/1
  If/1 -> If Action Subsystem/Action
  If/2 -> If Action Subsystem1/Action
  Selector1/1 -> If1/1
  Constant1/1 -> If1/2
  If1/1 -> If Action Subsystem2/Action
  [Index] -> If Action Subsystem/1(Index)
  [Index] -> If Action Subsystem1/1(In1)
  If1/2 -> If Action Subsystem3/Action
  [Index] -> If Action Subsystem2/1(Index)
  [Index] -> If Action Subsystem3/1(In1)

== system Mdl_Speed/Mdl_Speed_Task_sys/Digital_speed/Subsystem1/Interpolation&Trim_data/ADR_ECE ==
  Spd_Avg : Inport  OutDataTypeStr=uint16
  Action Port : ActionPort  ActionPortLabel=else
  Subsystem : Subsystem  TreatAsAtomicUnit=on  RTWFcnName=Interpolation_Other_Region
      settings: RTWFcnNameOpts=User specified
  Speed_ind : Outport  OutDataTypeStr=uint16  VectorParamsAs1DForOutWhenUnconnected=off
  wires:
  Spd_Avg/1 -> [Spd_Avg]
  [Spd_Avg] -> Subsystem/1(Spd_Avg)  "Spd_Avg"
  Subsystem/1(Interpolated_Data) -> Speed_ind/1

== system Mdl_Speed/Mdl_Speed_Task_sys/Digital_speed/Subsystem1/Interpolation&Trim_data/EUROPE_UK ==
  Spd_Avg : Inport  OutDataTypeStr=uint16
  Action Port : ActionPort  ActionPortLabel=elseif(u1 == u6|u1 == u7|u1==u8)
  Subsystem : Subsystem  TreatAsAtomicUnit=on  RTWFcnName=Interpolation_Other_Region
      settings: RTWFcnNameOpts=User specified
  Speed_ind : Outport  OutDataTypeStr=uint16  VectorParamsAs1DForOutWhenUnconnected=off
  wires:
  Spd_Avg/1 -> [Spd_Avg]
  [Spd_Avg] -> Subsystem/1(Spd_Avg)  "Spd_Avg"
  Subsystem/1(Interpolated_Data) -> Speed_ind/1

== system Mdl_Speed/Mdl_Speed_Task_sys/Digital_speed/Subsystem1/Interpolation&Trim_data/Subsystem ==
  Interpolated_data : Inport
  Data Store Read2 : DataStoreRead  DataStoreName=MCUID0262  IndexOptions=Index vector (dialog)  Indices=1  OutputSizes=1
  Data Store Read41 : DataStoreRead  DataStoreName=MCUID0262  IndexOptions=Index vector (dialog)  Indices=1  OutputSizes=1
  Less Than : RelationalOperator  Operator=<=  OutDataTypeStr=boolean  RndMeth=Floor  InputSameDT=off
  Speed_target_km : Subsystem  TreatAsAtomicUnit=on  RTWFcnName=Speed_target
      settings: RTWFcnNameOpts=User specified
  Speed_trimming_KM : Subsystem  TreatAsAtomicUnit=on  RTWFcnName=Speed_trimming
      settings: RTWFcnNameOpts=User specified
  Switch : Switch  Criteria=u2 ~= 0  SaturateOnIntegerOverflow=off  InputSameDT=off
  speed_internal_km : Subsystem
  speed_trim_km : Outport  VectorParamsAs1DForOutWhenUnconnected=off
  speed_trg : Outport  Port=2  VectorParamsAs1DForOutWhenUnconnected=off
  wires:
  Data Store Read41/1 -> Less Than/2
  [Speed_trim_km] -> speed_internal_km/1(speed_trim_km)
  Speed_trimming_KM/1(Speed_trim) -> speed_trim_km/1, [Speed_trim_km]
  Data Store Read2/1 -> Switch/3
  Switch/1 -> Speed_trimming_KM/1(speed_avg)  "Spd_Avg"
  speed_internal_km/1(speed_int_km) -> Speed_target_km/1(Speed_int)
  Speed_target_km/1(speed_trg) -> speed_trg/1
  Less Than/1 -> Switch/2
  Interpolated_data/1 -> Switch/1, Less Than/1

== system Mdl_Speed/Mdl_Speed_Task_sys/Digital_speed/Subsystem1/Interpolation&Trim_data/Subsystem1 ==
  note: kmtomiles_conversion
  Interpolated _Data : Inport
  Data Store Read2 : DataStoreRead  DataStoreName=MCUID0263  IndexOptions=Index vector (dialog)  Indices=1  OutputSizes=1
  Data Store Read41 : DataStoreRead  DataStoreName=MCUID0263  IndexOptions=Index vector (dialog)  Indices=1  OutputSizes=1
  Less Than : RelationalOperator  Operator=<=  OutDataTypeStr=boolean  RndMeth=Simplest  InputSameDT=off
  Speed_target_Miles : Subsystem  TreatAsAtomicUnit=on  RTWFcnName=Speed_target
      settings: RTWFcnNameOpts=User specified
  Speed_trimming_Miles : Subsystem  TreatAsAtomicUnit=on  RTWFcnName=Speed_trimming
      settings: RTWFcnNameOpts=User specified
  Switch : Switch  Criteria=u2 ~= 0  SaturateOnIntegerOverflow=off  InputSameDT=off
  kmtomiles_conversion1 : Subsystem
  speed_internal_Miles : Subsystem
  speed_trim2 : Outport  VectorParamsAs1DForOutWhenUnconnected=off
  speed_trg2 : Outport  Port=2  VectorParamsAs1DForOutWhenUnconnected=off
  wires:
  [Speed_trim] -> speed_internal_Miles/1(speed_trim)
  speed_internal_Miles/1(speed_int) -> Speed_target_Miles/1(Speed_int)
  Less Than/1 -> Switch/2
  Data Store Read41/1 -> Less Than/2
  Data Store Read2/1 -> Switch/3
  Switch/1 -> Speed_trimming_Miles/1(speed_avg)  "Spd_Avg2"
  Speed_trimming_Miles/1(Speed_trim) -> speed_trim2/1, [Speed_trim]
  kmtomiles_conversion1/1(speed_avg) -> Switch/1, Less Than/1
  Speed_target_Miles/1(speed_trg) -> speed_trg2/1
  Interpolated _Data/1 -> kmtomiles_conversion1/1(Input)

== system Mdl_Speed/Mdl_Speed_Task_sys/Digital_speed/Subsystem1/Interpolation&Trim_data/US_CAN_MAX ==
  spd_avg : Inport  OutDataTypeStr=uint16
  Action Port : ActionPort  ActionPortLabel=if(u1 == u2 | u1 == u3 |u1 == u4|u1==u5)
  Subsystem : Subsystem  TreatAsAtomicUnit=on  RTWFcnName=Interpolation_US_CANADA_MEXICO_Region
      settings: RTWSystemCode=Nonreusable function  RTWFcnNameOpts=User specified
  Speed_ind : Outport  OutDataTypeStr=uint16  VectorParamsAs1DForOutWhenUnconnected=off
  wires:
  spd_avg/1 -> [spd_avg]  "spd_avg"
  [spd_avg] -> Subsystem/1(Spd_Avg)  "speed_avg"
  Subsystem/1(Interpolated_Data) -> Speed_ind/1

== system Mdl_Speed/Mdl_Speed_Task_sys/Digital_speed/Subsystem1/Speed_Update_Time_and_Avg_check/Average_samples_km ==
  Input : Inport  OutDataTypeStr=uint32
  Speed_update_time : Inport  Port=2
  Speedtime_Update_Flag : Inport  Port=3
  Current_Sample_Count : Inport  Port=4
  Enable : EnablePort
  Cast : DataTypeConversion  OutDataTypeStr=uint16  SaturateOnIntegerOverflow=off  RndMeth=Floor
  Constant : Constant  Value=SPEED_ZERO  OutDataTypeStr=uint32
  Data Store Read : DataStoreRead  DataStoreName=Speedin_avg  IndexOptions=Index vector (dialog)  Indices=1  OutputSizes=1
  Data Store Write : DataStoreWrite  DataStoreName=Speedin_avg  IndexOptions=Index vector (dialog)  Indices=1  OutputSizes=1
  Data Store Write1 : DataStoreWrite  DataStoreName=l_Speedin_Collect  IndexOptions=Index vector (dialog)  Indices=1  OutputSizes=1
  Divide : Product  Inputs=*/  OutDataTypeStr=uint32  RndMeth=Simplest  SaturateOnIntegerOverflow=on
  Switch : Switch  Criteria=u2 ~= 0  SaturateOnIntegerOverflow=off  InputSameDT=off
  SP1_Average_km : Outport  OutDataTypeStr=uint16  VectorParamsAs1DForOutWhenUnconnected=off
  wires:
  Input/1 -> Divide/1
  Data Store Read/1 -> SP1_Average_km/1
  Divide/1 -> Cast/1
  Constant/1 -> Data Store Write1/1
  Cast/1 -> Data Store Write/1
  Speedtime_Update_Flag/1 -> Switch/2
  Current_Sample_Count/1 -> Switch/1
  Speed_update_time/1 -> Switch/3
  Switch/1 -> Divide/2

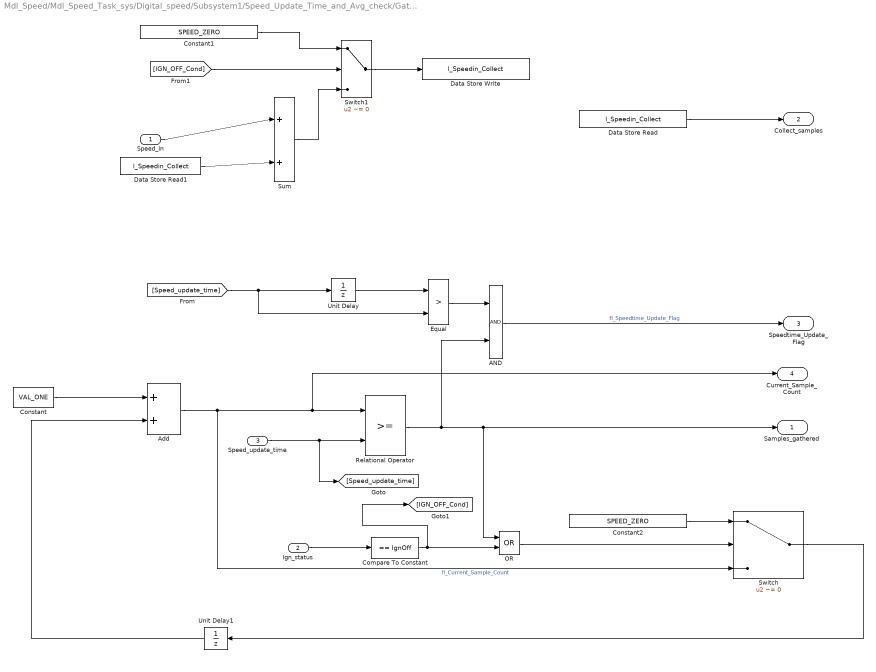
== system Mdl_Speed/Mdl_Speed_Task_sys/Digital_speed/Subsystem1/Speed_Update_Time_and_Avg_check/Gather_samples_km ==
  Speed_In : Inport  OutDataTypeStr=uint16
  Ign_status : Inport  Port=2  OutDataTypeStr=IgntionSubstateType
  Speed_update_time : Inport  Port=3
  AND : Logic  AllPortsSameDT=off  OutDataTypeStr=boolean
  Add : Sum  OutDataTypeStr=uint8  AccumDataTypeStr=uint8  RndMeth=Simplest
  Compare To Constant : simulink/Logic and Bit Operations/Compare To Constant  relop===  const=IgnOff  OutDataTypeStr=boolean
  Constant : Constant  Value=VAL_ONE  OutDataTypeStr=uint8
  Constant1 : Constant  Value=SPEED_ZERO  OutDataTypeStr=uint16
  Constant2 : Constant  Value=SPEED_ZERO  OutDataTypeStr=uint16
  Data Store Read : DataStoreRead  DataStoreName=l_Speedin_Collect  IndexOptions=Index vector (dialog)  Indices=1  OutputSizes=1
  Data Store Read1 : DataStoreRead  DataStoreName=l_Speedin_Collect  IndexOptions=Index vector (dialog)  Indices=1  OutputSizes=1
  Data Store Write : DataStoreWrite  DataStoreName=l_Speedin_Collect  IndexOptions=Index vector (dialog)  Indices=1  OutputSizes=1
  Equal : RelationalOperator  Operator=>  OutDataTypeStr=boolean  RndMeth=Simplest  InputSameDT=off
  OR : Logic  Operator=OR  AllPortsSameDT=off  OutDataTypeStr=boolean
  Relational Operator : RelationalOperator  OutDataTypeStr=boolean  RndMeth=Simplest  InputSameDT=off
  Sum : Sum  Inputs=|++  AccumDataTypeStr=uint32
  Switch : Switch  Criteria=u2 ~= 0  SaturateOnIntegerOverflow=off  InputSameDT=off
  Switch1 : Switch  Criteria=u2 ~= 0  SaturateOnIntegerOverflow=off  InputSameDT=off
  Unit Delay : UnitDelay  SampleTime=-1  StateName=l_Prev_Speed_Update_Time  HasFrameUpgradeWarning=on
  Unit Delay1 : UnitDelay  SampleTime=-1  StateName=Speed_index_count  HasFrameUpgradeWarning=on
  Samples_gathered : Outport  OutDataTypeStr=boolean  VectorParamsAs1DForOutWhenUnconnected=off
  Collect_samples : Outport  Port=2  OutDataTypeStr=uint32  VectorParamsAs1DForOutWhenUnconnected=off
  Speedtime_Update_Flag : Outport  Port=3  VectorParamsAs1DForOutWhenUnconnected=off
  Current_Sample_Count : Outport  Port=4  VectorParamsAs1DForOutWhenUnconnected=off
  wires:
  Speed_update_time/1 -> [Speed_update_time], Relational Operator/2
  Unit Delay1/1 -> Add/2
  Constant/1 -> Add/1
  Constant2/1 -> Switch/1
  Switch/1 -> Unit Delay1/1
  Add/1 -> Current_Sample_Count/1, Relational Operator/1, Switch/3  "fl_Current_Sample_Count"
  Ign_status/1 -> Compare To Constant/1
  Data Store Read/1 -> Collect_samples/1
  OR/1 -> Switch/2
  Compare To Constant/1 -> [IGN_OFF_Cond], OR/2
  Data Store Read1/1 -> Sum/2
  Speed_In/1 -> Sum/1
  [Speed_update_time] -> Unit Delay/1, Equal/2
  Unit Delay/1 -> Equal/1
  Equal/1 -> AND/1
  Relational Operator/1 -> OR/1, Samples_gathered/1, AND/2
  AND/1 -> Speedtime_Update_Flag/1  "fl_Speedtime_Update_Flag"
  [IGN_OFF_Cond] -> Switch1/2
  Sum/1 -> Switch1/3
  Switch1/1 -> Data Store Write/1
  Constant1/1 -> Switch1/1

== system Mdl_Speed/Mdl_Speed_Task_sys/Digital_speed/Subsystem2/For Iterator Subsystem/If Action Subsystem ==
  Index : Inport
  Action Port : ActionPort
  Chart : Stateflow chart  TreatAsAtomicUnit=on
  Constant : Constant  Value=Initial_data
  wires:
  Constant/1 -> Chart/1(Initial_data)
  Index/1 -> Chart/2(Index)

== system Mdl_Speed/Mdl_Speed_Task_sys/Digital_speed/Subsystem2/For Iterator Subsystem/If Action Subsystem1 ==
  In1 : Inport
  Action Port : ActionPort
  Chart : Stateflow chart  TreatAsAtomicUnit=on
  wires:
  In1/1 -> Chart/1(Index)

== system Mdl_Speed/Mdl_Speed_Task_sys/Digital_speed/Subsystem2/For Iterator Subsystem/If Action Subsystem2 ==
  Index : Inport
  Action Port : ActionPort
  Chart : Stateflow chart  TreatAsAtomicUnit=on
  Constant : Constant  Value=Initial_data
  wires:
  Constant/1 -> Chart/1(Initial_data)
  Index/1 -> Chart/2(Index)

== system Mdl_Speed/Mdl_Speed_Task_sys/Digital_speed/Subsystem2/For Iterator Subsystem/If Action Subsystem3 ==
  In1 : Inport
  Action Port : ActionPort
  Chart : Stateflow chart  TreatAsAtomicUnit=on
  wires:
  In1/1 -> Chart/1(Index)

== system Mdl_Speed/Mdl_Speed_Task_sys/Digital_speed/Subsystem1/Interpolation&Trim_data/ADR_ECE/Subsystem ==
  Spd_Avg : Inport
  Constant4 : Constant  Value=SPEED_AVG_REF
  Data Store Read : DataStoreRead  DataStoreName=DSpeed_Int_Ref_Other  IndexOptions=Index vector (dialog)  Indices=1  OutputSizes=1
  Lookup Table Dynamic : simulink/Lookup Tables/Lookup Table Dynamic  LookUpMeth=Interpolation-Use End Values  OutDataType=fixdt('uint16')  OutScaling=[]  OutputDataTypeScalingMode=Specify via dialog  OutDataTypeStr=uint16  RndMeth=Simplest  DoSatur=off
  Interpolated_Data : Outport  VectorParamsAs1DForOutWhenUnconnected=off
  wires:
  Spd_Avg/1 -> Lookup Table Dynamic/1
  Constant4/1 -> Lookup Table Dynamic/2
  Data Store Read/1 -> Lookup Table Dynamic/3
  Lookup Table Dynamic/1 -> Interpolated_Data/1

== system Mdl_Speed/Mdl_Speed_Task_sys/Digital_speed/Subsystem1/Interpolation&Trim_data/EUROPE_UK/Subsystem ==
  Spd_Avg : Inport
  Constant4 : Constant  Value=SPEED_AVG_REF
  Data Store Read : DataStoreRead  DataStoreName=DSpeed_Int_Ref_Other  IndexOptions=Index vector (dialog)  Indices=1  OutputSizes=1
  Lookup Table Dynamic : simulink/Lookup Tables/Lookup Table Dynamic  LookUpMeth=Interpolation-Use End Values  OutDataType=fixdt('uint16')  OutScaling=[]  OutputDataTypeScalingMode=Specify via dialog  OutDataTypeStr=uint16  RndMeth=Simplest  DoSatur=off
  Interpolated_Data : Outport  VectorParamsAs1DForOutWhenUnconnected=off
  wires:
  Spd_Avg/1 -> Lookup Table Dynamic/1
  Constant4/1 -> Lookup Table Dynamic/2
  Data Store Read/1 -> Lookup Table Dynamic/3
  Lookup Table Dynamic/1 -> Interpolated_Data/1

== system Mdl_Speed/Mdl_Speed_Task_sys/Digital_speed/Subsystem1/Interpolation&Trim_data/Subsystem/Speed_target_km ==
  Speed_int : Inport
  Constant2 : Constant  Value=RESOLUTION_VAL_100  OutDataTypeStr=uint16
  Constant3 : Constant  Value=RESOLUTION_VAL_100  OutDataTypeStr=uint16
  Divide : Product  Inputs=*/  SaturateOnIntegerOverflow=on
  If : If  IfExpression=u1 < 50
  If Action Subsystem : Subsystem  TreatAsAtomicUnit=on
  If Action Subsystem1 : Subsystem  TreatAsAtomicUnit=on
  Merge : Merge
  Mod : Math  Operator=mod  SignedPower=on
  speed_trg : Outport  VectorParamsAs1DForOutWhenUnconnected=off
  wires:
  Divide/1 -> If Action Subsystem1/1(In1), If Action Subsystem/1(In1)
  Constant3/1 -> Divide/2
  If/1 -> If Action Subsystem/Action
  [Speed_int] -> Divide/1
  If Action Subsystem1/1(Out1) -> Merge/2
  Merge/1 -> speed_trg/1
  [Speed_int] -> Mod/1
  Mod/1 -> If/1
  If/2 -> If Action Subsystem1/Action
  Constant2/1 -> Mod/2
  If Action Subsystem/1(Out1) -> Merge/1
  Speed_int/1 -> [Speed_int]
